simulink model "M4B11_modified_AGC_PI_constant_power"  (R2024b)
settings: Solver=VariableStepAuto  StartTime=0.0  StopTime=100  RelTol=1e-3
InitFcn:
  | clear;
  | load('parameterinit.mat');
  | set_param('M4B11_modified_AGC_PI_constant_power/Python2Sim2','value','[0 0]');
  | acom=100;
  | bcom=50;
  | lam=100;
values from neighbouring files (symbols this model uses):
  ACgirdinit =     [datainit.mat]    (also in parameterinit.mat)
  AVm0 = [11.3576294988 11.3576294988]    [datainit.mat]    (also in parameterinit.mat)
  commun = [1 1 1 0]    [datainit.mat]    (also in initAll.m = [1,1,1,0]; parameterinit.mat)
  DataDelay = [0  0; 0  0; 0  0; 0  0]    [datainit.mat]    (also in initAll.m = 0.0*DataDelay; parameterinit.mat)
  ESinit =     [datainit.mat]    (also in parameterinit.mat)
  fB = 50    [datainit.mat]    (also in initAll.m; parameterinit.mat)
  Geninit =     [datainit.mat]    (also in initAll.m = Generator_init(opdata,SynMach_in_gidx); parameterinit.mat)
  SgridB = 100    [datainit.mat]    (also in initAll.m = resultsac.baseMVA; parameterinit.mat)
  wB = 314.159265359    [datainit.mat]    (also in initAll.m; parameterinit.mat)
  Windinit =     [datainit.mat]    (also in parameterinit.mat)
undefined symbols (not defined in the file or in its folder): c1, c2, c3, c4, c5, c6, cp_nom, lambda_nom, Loadinit, P_wind_base, Pelec_base, Pnom
libraries: spsBistableLib x9, slpidlib x2, simulink_extras x2
(part 3 of 5)

== system M4B11_modified_AGC_PI_constant_power/ES1/ control1 ==
  usdq : Inport
  isdq : Inport  Port=2
  delta : Inport  Port=3
  Enable : EnablePort
  Add : Sum  Inputs=|-+
  Add2 : Sum  Inputs=|-+
  Add3 : Sum
  Add4 : Sum  Inputs=-+
  Add6 : Sum  Inputs=|++
  Add7 : Sum  Inputs=+-
  Complex to Magnitude-Angle : ComplexToMagnitudeAngle
  Complex to Real-Imag1 : ComplexToRealImag
  Constant : Constant
  Constant1 : Constant  Value=usd0
  Constant2 : Constant  Value=0
  Constant3 : Constant  Value=Q0
  Constant4 : Constant
  Demux : Demux  Outputs=2
  Demux1 : Demux  Outputs=2
  Gain : Gain  Gain=0.01
  Gain1 : Gain  Gain=-1
  K5 : Gain  Gain=Lpr  SaturateOnIntegerOverflow=on  OutDataTypeStr=Inherit: Same as input  ParamDataTypeStr=Inherit: Same as input
  K6 : Gain  Gain=Lpr  SaturateOnIntegerOverflow=on  OutDataTypeStr=Inherit: Same as input  ParamDataTypeStr=Inherit: Same as input
  Magnitude-Angle to Complex : MagnitudeAngleToComplex
  Product{1,4..6} (4 alike) : Product  RndMeth=Zero
  Real-Imag to Complex : RealImagToComplex
  Scope : Scope
  Scope1 : Scope
  Scope2 : Scope  NumInputPorts=2
  Scope3 : Scope  NumInputPorts=2
  Scope7 : Scope  NumInputPorts=2
  Sum : Sum  Inputs=|+-
  Sum2 : Sum  Inputs=|+-  SaturateOnIntegerOverflow=on
  Sum23 : Sum  Inputs=|+-  SaturateOnIntegerOverflow=on
  Sum9 : Sum  Inputs=|+-  SaturateOnIntegerOverflow=on
  control_AC_voltage : Subsystem  VariantControl=VSC1q_Variant2
  control_AC_voltage1 : Subsystem  VariantControl=VSC1q_Variant2
  in_D_PI : Subsystem  mask{KP_=KpId_VSC_A, KI_=KiId_VSC_A, Upper_limit=inf, Lower_limit=-inf, Upper_saturation_limit=inf, Lower_saturation_limit=-inf, integrator_init=Md_A_0}
      mask prompts: KP_ "比例系数P"; KI_ "积分系数I"; Upper_limit "限幅上限"; Lower_limit "限幅下限"; Upper_saturation_limit "积分饱和上限"; Lower_saturation_limit "积分饱和下限"; integrator_init "积分初始值"
      mask DialogControl Container4 Prompt: 控制参数
      mask DialogControl Container5 Prompt: 初始值
      mask Display: disp('PI')
  in_Q_PI : Subsystem  mask{KP_=KpIq_VSC_A, KI_=KiIq_VSC_A, Upper_limit=inf, Lower_limit=-inf, Upper_saturation_limit=inf, Lower_saturation_limit=-inf, integrator_init=Mq_A_0}
      mask prompts: KP_ "比例系数P"; KI_ "积分系数I"; Upper_limit "限幅上限"; Lower_limit "限幅下限"; Upper_saturation_limit "积分饱和上限"; Lower_saturation_limit "积分饱和下限"; integrator_init "积分初始值"
      mask DialogControl Container4 Prompt: 控制参数
      mask DialogControl Container5 Prompt: 初始值
      mask Display: disp('PI')
  ucx : Outport
  ucy : Outport  Port=2
  wires:
  Magnitude-Angle to Complex/1 -> Complex to Real-Imag1/1
  Add/1 -> Real-Imag to Complex/2
  Add2/1 -> Real-Imag to Complex/1
  delta/1 -> Add6/2
  Add6/1 -> Magnitude-Angle to Complex/2
  Complex to Magnitude-Angle/2 -> Add6/1
  Sum9/1 -> in_D_PI/1(In1)
  K5/1 -> Add3/1
  [usd] -> Add3/2
  Add3/1 -> Add2/2
  in_D_PI/1(Out1) -> Add2/1
  Constant/1 -> Product4/2
  [isq] -> Product4/1
  [isd] -> Scope7/2, Sum9/2
  Product4/1 -> K5/1
  Demux1/1 -> [isd]
  Demux/1 -> [usd]
  Demux1/2 -> [isq]
  Demux/2 -> [usq]
  isdq/1 -> Demux1/1
  usdq/1 -> Demux/1
  [usq] -> Add4/2
  K6/1 -> Add4/1
  in_Q_PI/1(Out1) -> Add/1
  Sum23/1 -> in_Q_PI/1(In1)
  [isd] -> Product1/1
  [isq] -> Sum23/2, Scope3/2
  Product1/1 -> K6/1
  Constant4/1 -> Product1/2
  Add4/1 -> Add/2
  Real-Imag to Complex/1 -> Complex to Magnitude-Angle/1
  Complex to Magnitude-Angle/1 -> Magnitude-Angle to Complex/1
  Complex to Real-Imag1/1 -> ucx/1
  Complex to Real-Imag1/2 -> ucy/1
  [usd] -> Scope1/1, control_AC_voltage/1(usd)
  control_AC_voltage/1(isdref) -> Scope7/1, Sum9/1
  [isq] -> Product5/2
  Product5/1 -> Add7/2
  [usd] -> Product5/1
  [isd] -> Product6/2
  Product6/1 -> Add7/1
  [usq] -> Product6/1
  Gain/1 -> Sum/2
  control_AC_voltage1/1(isqref) -> Scope3/1, Sum23/1
  [usq] -> Scope2/1, control_AC_voltage1/1(usq)
  Constant2/1 -> Scope2/2, control_AC_voltage1/2(usqref)
  Add7/1 -> Scope/1, Gain1/1
  Sum2/1 -> Gain/1
  Constant3/1 -> Sum2/2
  Gain1/1 -> Sum2/1
  Sum/1 -> control_AC_voltage/2(usdref)
  Constant1/1 -> Sum/1

== system M4B11_modified_AGC_PI_constant_power/ES1/in_D_PI ==
  In1 : Inport
  Ki : Gain  Gain=KI_  SaturateOnIntegerOverflow=on  OutDataTypeStr=Inherit: Same as input  ParamDataTypeStr=Inherit: Same as input
  Kp : Gain  Gain=KP_  SaturateOnIntegerOverflow=on  OutDataTypeStr=Inherit: Same as input  ParamDataTypeStr=Inherit: Same as input
  Saturation2 : Saturate  UpperLimit=Upper_limit  LowerLimit=Lower_limit
  Sum12 : Sum  SaturateOnIntegerOverflow=on
  integrator : Integrator  InitialCondition=integrator_init  LimitOutput=on  UpperSaturationLimit=Upper_saturation_limit  LowerSaturationLimit=Lower_saturation_limit
  Out1 : Outport
  wires:
  In1/1 -> Ki/1, Kp/1
  Kp/1 -> Sum12/2
  Ki/1 -> integrator/1
  integrator/1 -> Sum12/1
  Saturation2/1 -> Out1/1
  Sum12/1 -> Saturation2/1

== system M4B11_modified_AGC_PI_constant_power/ES1/output ==
  is_xy : Inport
  Pe : Inport  Port=2
  Brecx : Constant  Value=0
  Brecy : Constant  Value=0
  Bus Creator : BusCreator  Inputs=4
  Constant : Constant
  Gain : Gain  Gain=SvscB./SgridB
  Gain1 : Gain  Gain=-1
  Gain2 : Gain  Gain=-1
  Gain6 : Gain
  Grecx : Constant  Value=0
  Grecy : Constant  Value=0
  Mux3 : Mux
  Sum : Sum  Inputs=|++
  m : Outport
  isxy : Outport  Port=2
  GBxy : Outport  Port=3
  wires:
  Bus Creator/1 -> m/1
  Gain6/1 -> GBxy/1, Bus Creator/4  "GBxy"
  Mux3/1 -> Gain6/1
  Grecx/1 -> Mux3/1
  Brecx/1 -> Mux3/3
  Grecy/1 -> Mux3/2
  Brecy/1 -> Mux3/4
  Gain1/1 -> isxy/1, Bus Creator/1  "is_xy"
  Gain2/1 -> Bus Creator/2  "Pe"
  Gain/1 -> Gain1/1  "is_xy"
  Pe/1 -> Gain2/1  "Pe"
  [WreES1] -> Sum/1  "Pe"
  Constant/1 -> Sum/2
  Sum/1 -> Bus Creator/3  "w"
  is_xy/1 -> Gain/1

== system M4B11_modified_AGC_PI_constant_power/ES1/xy->dq ==
  Ixy : Inport
  Theta : Inport  Port=2
  Complex to Magnitude-Angle : ComplexToMagnitudeAngle
  Complex to Real-Imag : ComplexToRealImag
  Demux1 : Demux  Outputs=2
      settings: DisplayOption=none
  Magnitude-Angle to Complex : MagnitudeAngleToComplex
  Mux : Mux  Inputs=2
  Real-Imag to Complex : RealImagToComplex
  Scope : Scope
  Scope1 : Scope
  Sum1 : Sum  Inputs=|+-  SaturateOnIntegerOverflow=on
  Idq : Outport
  wires:
  Complex to Magnitude-Angle/1 -> Magnitude-Angle to Complex/1
  Theta/1 -> Sum1/2
  Complex to Magnitude-Angle/2 -> Sum1/1, Scope1/1
  Demux1/1 -> Real-Imag to Complex/1
  Complex to Real-Imag/2 -> Mux/2  "Iq"
  Mux/1 -> Idq/1
  Complex to Real-Imag/1 -> Mux/1  "Id"
  Magnitude-Angle to Complex/1 -> Complex to Real-Imag/1
  Sum1/1 -> Magnitude-Angle to Complex/2, Scope/1
  Demux1/2 -> Real-Imag to Complex/2
  Real-Imag to Complex/1 -> Complex to Magnitude-Angle/1
  Ixy/1 -> Demux1/1

== system M4B11_modified_AGC_PI_constant_power/ES2/ control1 ==
  usdq : Inport
  isdq : Inport  Port=2
  delta : Inport  Port=3
  Enable : EnablePort
  Add : Sum  Inputs=|-+
  Add2 : Sum  Inputs=|-+
  Add3 : Sum
  Add4 : Sum  Inputs=-+
  Add6 : Sum  Inputs=|++
  Add7 : Sum  Inputs=+-
  Complex to Magnitude-Angle : ComplexToMagnitudeAngle
  Complex to Real-Imag1 : ComplexToRealImag
  Constant : Constant
  Constant1 : Constant  Value=usd0
  Constant2 : Constant  Value=0
  Constant3 : Constant  Value=Q0
  Constant4 : Constant
  Demux : Demux  Outputs=2
  Demux1 : Demux  Outputs=2
  Gain : Gain  Gain=0.01
  Gain1 : Gain  Gain=-1
  K5 : Gain  Gain=Lpr  SaturateOnIntegerOverflow=on  OutDataTypeStr=Inherit: Same as input  ParamDataTypeStr=Inherit: Same as input
  K6 : Gain  Gain=Lpr  SaturateOnIntegerOverflow=on  OutDataTypeStr=Inherit: Same as input  ParamDataTypeStr=Inherit: Same as input
  Magnitude-Angle to Complex : MagnitudeAngleToComplex
  Product{1,4..6} (4 alike) : Product  RndMeth=Zero
  Real-Imag to Complex : RealImagToComplex
  Scope{,1..2,7} (4 alike) : Scope
  Sum : Sum  Inputs=|+-
  Sum2 : Sum  Inputs=|+-  SaturateOnIntegerOverflow=on
  Sum23 : Sum  Inputs=|+-  SaturateOnIntegerOverflow=on
  Sum9 : Sum  Inputs=|+-  SaturateOnIntegerOverflow=on
  control_AC_voltage : Subsystem  VariantControl=VSC1q_Variant2
  control_AC_voltage1 : Subsystem  VariantControl=VSC1q_Variant2
  in_D_PI : Subsystem  mask{KP_=KpId_VSC_A, KI_=KiId_VSC_A, Upper_limit=inf, Lower_limit=-inf, Upper_saturation_limit=inf, Lower_saturation_limit=-inf, integrator_init=Md_A_0}
      mask prompts: KP_ "比例系数P"; KI_ "积分系数I"; Upper_limit "限幅上限"; Lower_limit "限幅下限"; Upper_saturation_limit "积分饱和上限"; Lower_saturation_limit "积分饱和下限"; integrator_init "积分初始值"
      mask DialogControl Container4 Prompt: 控制参数
      mask DialogControl Container5 Prompt: 初始值
      mask Display: disp('PI')
  in_Q_PI : Subsystem  mask{KP_=KpIq_VSC_A, KI_=KiIq_VSC_A, Upper_limit=inf, Lower_limit=-inf, Upper_saturation_limit=inf, Lower_saturation_limit=-inf, integrator_init=Mq_A_0}
      mask prompts: KP_ "比例系数P"; KI_ "积分系数I"; Upper_limit "限幅上限"; Lower_limit "限幅下限"; Upper_saturation_limit "积分饱和上限"; Lower_saturation_limit "积分饱和下限"; integrator_init "积分初始值"
      mask DialogControl Container4 Prompt: 控制参数
      mask DialogControl Container5 Prompt: 初始值
      mask Display: disp('PI')
  ucx : Outport
  ucy : Outport  Port=2
  wires:
  Magnitude-Angle to Complex/1 -> Complex to Real-Imag1/1
  Add/1 -> Real-Imag to Complex/2
  Add2/1 -> Real-Imag to Complex/1
  delta/1 -> Add6/2
  Add6/1 -> Magnitude-Angle to Complex/2
  Complex to Magnitude-Angle/2 -> Add6/1
  Sum9/1 -> in_D_PI/1(In1)
  K5/1 -> Add3/1
  [usd] -> Add3/2
  Add3/1 -> Add2/2
  in_D_PI/1(Out1) -> Add2/1
  Constant/1 -> Product4/2
  [isq] -> Product4/1
  [isd] -> Sum9/2
  Product4/1 -> K5/1
  Demux1/1 -> [isd]
  Demux/1 -> [usd]
  Demux1/2 -> [isq]
  Demux/2 -> [usq]
  isdq/1 -> Demux1/1
  usdq/1 -> Demux/1
  [usq] -> Add4/2
  K6/1 -> Add4/1
  in_Q_PI/1(Out1) -> Add/1
  Sum23/1 -> in_Q_PI/1(In1)
  [isd] -> Product1/1
  [isq] -> Sum23/2
  Product1/1 -> K6/1
  Constant4/1 -> Product1/2
  Add4/1 -> Add/2
  Real-Imag to Complex/1 -> Complex to Magnitude-Angle/1
  Complex to Magnitude-Angle/1 -> Magnitude-Angle to Complex/1
  Complex to Real-Imag1/1 -> ucx/1
  Complex to Real-Imag1/2 -> ucy/1
  [usd] -> Scope1/1, control_AC_voltage/1(usd)
  control_AC_voltage/1(isdref) -> Scope7/1, Sum9/1
  [isq] -> Product5/2
  Product5/1 -> Add7/2
  [usd] -> Product5/1
  [isd] -> Product6/2
  Product6/1 -> Add7/1
  [usq] -> Product6/1
  Gain/1 -> Sum/2
  control_AC_voltage1/1(isqref) -> Sum23/1
  [usq] -> Scope2/1, control_AC_voltage1/1(usq)
  Constant2/1 -> control_AC_voltage1/2(usqref)
  Add7/1 -> Scope/1, Gain1/1
  Sum2/1 -> Gain/1
  Constant3/1 -> Sum2/2
  Gain1/1 -> Sum2/1
  Sum/1 -> control_AC_voltage/2(usdref)
  Constant1/1 -> Sum/1

== system M4B11_modified_AGC_PI_constant_power/ES2/output ==
  is_xy : Inport
  Pe : Inport  Port=2
  Brecx : Constant  Value=0
  Brecy : Constant  Value=0
  Bus Creator : BusCreator  Inputs=4
  Constant : Constant
  Gain : Gain  Gain=SvscB./SgridB
  Gain1 : Gain  Gain=-1
  Gain2 : Gain  Gain=-1
  Gain6 : Gain
  Grecx : Constant  Value=0
  Grecy : Constant  Value=0
  Mux3 : Mux
  Sum : Sum  Inputs=|++
  m : Outport
  isxy : Outport  Port=2
  GBxy : Outport  Port=3
  wires:
  Bus Creator/1 -> m/1
  Gain6/1 -> GBxy/1, Bus Creator/4  "GBxy"
  Mux3/1 -> Gain6/1
  Grecx/1 -> Mux3/1
  Brecx/1 -> Mux3/3
  Grecy/1 -> Mux3/2
  Brecy/1 -> Mux3/4
  Gain1/1 -> isxy/1, Bus Creator/1  "is_xy"
  Gain2/1 -> Bus Creator/2  "Pe"
  Gain/1 -> Gain1/1  "is_xy"
  Pe/1 -> Gain2/1  "Pe"
  Constant/1 -> Sum/2
  [WreES2] -> Sum/1  "Pe"
  Sum/1 -> Bus Creator/3  "w"
  is_xy/1 -> Gain/1

== system M4B11_modified_AGC_PI_constant_power/ES2/xy->dq ==
  Ixy : Inport
  Theta : Inport  Port=2
  Complex to Magnitude-Angle : ComplexToMagnitudeAngle
  Complex to Real-Imag : ComplexToRealImag
  Demux1 : Demux  Outputs=2
      settings: DisplayOption=none
  Magnitude-Angle to Complex : MagnitudeAngleToComplex
  Mux : Mux  Inputs=2
  Real-Imag to Complex : RealImagToComplex
  Scope : Scope
  Scope1 : Scope
  Sum1 : Sum  Inputs=|+-  SaturateOnIntegerOverflow=on
  Idq : Outport
  wires:
  Complex to Magnitude-Angle/1 -> Magnitude-Angle to Complex/1
  Theta/1 -> Sum1/2
  Complex to Magnitude-Angle/2 -> Sum1/1, Scope1/1
  Demux1/1 -> Real-Imag to Complex/1
  Complex to Real-Imag/2 -> Mux/2  "Iq"
  Mux/1 -> Idq/1
  Complex to Real-Imag/1 -> Mux/1  "Id"
  Magnitude-Angle to Complex/1 -> Complex to Real-Imag/1
  Sum1/1 -> Magnitude-Angle to Complex/2, Scope/1
  Demux1/2 -> Real-Imag to Complex/2
  Real-Imag to Complex/1 -> Complex to Magnitude-Angle/1
  Ixy/1 -> Demux1/1

== system M4B11_modified_AGC_PI_constant_power/ES3/ control1 ==
  usdq : Inport
  isdq : Inport  Port=2
  delta : Inport  Port=3
  Enable : EnablePort
  Add : Sum  Inputs=|-+
  Add2 : Sum  Inputs=|-+
  Add3 : Sum
  Add4 : Sum  Inputs=-+
  Add6 : Sum  Inputs=|++
  Add7 : Sum  Inputs=+-
  Complex to Magnitude-Angle : ComplexToMagnitudeAngle
  Complex to Real-Imag1 : ComplexToRealImag
  Constant : Constant
  Constant1 : Constant  Value=usd0
  Constant2 : Constant  Value=0
  Constant3 : Constant  Value=Q0
  Constant4 : Constant
  Demux : Demux  Outputs=2
  Demux1 : Demux  Outputs=2
  Gain : Gain  Gain=0.01
  Gain1 : Gain  Gain=-1
  K5 : Gain  Gain=Lpr  SaturateOnIntegerOverflow=on  OutDataTypeStr=Inherit: Same as input  ParamDataTypeStr=Inherit: Same as input
  K6 : Gain  Gain=Lpr  SaturateOnIntegerOverflow=on  OutDataTypeStr=Inherit: Same as input  ParamDataTypeStr=Inherit: Same as input
  Magnitude-Angle to Complex : MagnitudeAngleToComplex
  Product{1,4..6} (4 alike) : Product  RndMeth=Zero
  Real-Imag to Complex : RealImagToComplex
  Scope{,1..2,7} (4 alike) : Scope
  Sum : Sum  Inputs=|+-
  Sum2 : Sum  Inputs=|+-  SaturateOnIntegerOverflow=on
  Sum23 : Sum  Inputs=|+-  SaturateOnIntegerOverflow=on
  Sum9 : Sum  Inputs=|+-  SaturateOnIntegerOverflow=on
  control_AC_voltage : Subsystem  VariantControl=VSC1q_Variant2
  control_AC_voltage1 : Subsystem  VariantControl=VSC1q_Variant2
  in_D_PI : Subsystem  mask{KP_=KpId_VSC_A, KI_=KiId_VSC_A, Upper_limit=inf, Lower_limit=-inf, Upper_saturation_limit=inf, Lower_saturation_limit=-inf, integrator_init=Md_A_0}
      mask prompts: KP_ "比例系数P"; KI_ "积分系数I"; Upper_limit "限幅上限"; Lower_limit "限幅下限"; Upper_saturation_limit "积分饱和上限"; Lower_saturation_limit "积分饱和下限"; integrator_init "积分初始值"
      mask DialogControl Container4 Prompt: 控制参数
      mask DialogControl Container5 Prompt: 初始值
      mask Display: disp('PI')
  in_Q_PI : Subsystem  mask{KP_=KpIq_VSC_A, KI_=KiIq_VSC_A, Upper_limit=inf, Lower_limit=-inf, Upper_saturation_limit=inf, Lower_saturation_limit=-inf, integrator_init=Mq_A_0}
      mask prompts: KP_ "比例系数P"; KI_ "积分系数I"; Upper_limit "限幅上限"; Lower_limit "限幅下限"; Upper_saturation_limit "积分饱和上限"; Lower_saturation_limit "积分饱和下限"; integrator_init "积分初始值"
      mask DialogControl Container4 Prompt: 控制参数
      mask DialogControl Container5 Prompt: 初始值
      mask Display: disp('PI')
  ucx : Outport
  ucy : Outport  Port=2
  wires:
  Magnitude-Angle to Complex/1 -> Complex to Real-Imag1/1
  Add/1 -> Real-Imag to Complex/2
  Add2/1 -> Real-Imag to Complex/1
  delta/1 -> Add6/2
  Add6/1 -> Magnitude-Angle to Complex/2
  Complex to Magnitude-Angle/2 -> Add6/1
  Sum9/1 -> in_D_PI/1(In1)
  K5/1 -> Add3/1
  [usd] -> Add3/2
  Add3/1 -> Add2/2
  in_D_PI/1(Out1) -> Add2/1
  Constant/1 -> Product4/2
  [isq] -> Product4/1
  [isd] -> Sum9/2
  Product4/1 -> K5/1
  Demux1/1 -> [isd]
  Demux/1 -> [usd]
  Demux1/2 -> [isq]
  Demux/2 -> [usq]
  isdq/1 -> Demux1/1
  usdq/1 -> Demux/1
  [usq] -> Add4/2
  K6/1 -> Add4/1
  in_Q_PI/1(Out1) -> Add/1
  Sum23/1 -> in_Q_PI/1(In1)
  [isd] -> Product1/1
  [isq] -> Sum23/2
  Product1/1 -> K6/1
  Constant4/1 -> Product1/2
  Add4/1 -> Add/2
  Real-Imag to Complex/1 -> Complex to Magnitude-Angle/1
  Complex to Magnitude-Angle/1 -> Magnitude-Angle to Complex/1
  Complex to Real-Imag1/1 -> ucx/1
  Complex to Real-Imag1/2 -> ucy/1
  [usd] -> Scope1/1, control_AC_voltage/1(usd)
  control_AC_voltage/1(isdref) -> Scope7/1, Sum9/1
  [isq] -> Product5/2
  Product5/1 -> Add7/2
  [usd] -> Product5/1
  [isd] -> Product6/2
  Product6/1 -> Add7/1
  [usq] -> Product6/1
  Gain/1 -> Sum/2
  control_AC_voltage1/1(isqref) -> Sum23/1
  [usq] -> Scope2/1, control_AC_voltage1/1(usq)
  Constant2/1 -> control_AC_voltage1/2(usqref)
  Add7/1 -> Scope/1, Gain1/1
  Sum2/1 -> Gain/1
  Constant3/1 -> Sum2/2
  Gain1/1 -> Sum2/1
  Sum/1 -> control_AC_voltage/2(usdref)
  Constant1/1 -> Sum/1

== system M4B11_modified_AGC_PI_constant_power/ES3/in_D_PI ==
  In1 : Inport
  Ki : Gain  Gain=KI_  SaturateOnIntegerOverflow=on  OutDataTypeStr=Inherit: Same as input  ParamDataTypeStr=Inherit: Same as input
  Kp : Gain  Gain=KP_  SaturateOnIntegerOverflow=on  OutDataTypeStr=Inherit: Same as input  ParamDataTypeStr=Inherit: Same as input
  Saturation2 : Saturate  UpperLimit=Upper_limit  LowerLimit=Lower_limit
  Sum12 : Sum  SaturateOnIntegerOverflow=on
  integrator : Integrator  InitialCondition=integrator_init  LimitOutput=on  UpperSaturationLimit=Upper_saturation_limit  LowerSaturationLimit=Lower_saturation_limit
  Out1 : Outport
  wires:
  In1/1 -> Ki/1, Kp/1
  Kp/1 -> Sum12/2
  Ki/1 -> integrator/1
  integrator/1 -> Sum12/1
  Saturation2/1 -> Out1/1
  Sum12/1 -> Saturation2/1

== system M4B11_modified_AGC_PI_constant_power/ES3/output ==
  is_xy : Inport
  Pe : Inport  Port=2
  Brecx : Constant  Value=0
  Brecy : Constant  Value=0
  Bus Creator : BusCreator  Inputs=4
  Constant : Constant
  Gain : Gain  Gain=SvscB./SgridB
  Gain1 : Gain  Gain=-1
  Gain2 : Gain  Gain=-1
  Gain6 : Gain
  Grecx : Constant  Value=0
  Grecy : Constant  Value=0
  Mux3 : Mux
  Sum : Sum  Inputs=|++
  m : Outport
  isxy : Outport  Port=2
  GBxy : Outport  Port=3
  wires:
  Bus Creator/1 -> m/1
  Gain6/1 -> GBxy/1, Bus Creator/4  "GBxy"
  Mux3/1 -> Gain6/1
  Grecx/1 -> Mux3/1
  Brecx/1 -> Mux3/3
  Grecy/1 -> Mux3/2
  Brecy/1 -> Mux3/4
  Gain1/1 -> isxy/1, Bus Creator/1  "is_xy"
  Gain2/1 -> Bus Creator/2  "Pe"
  Gain/1 -> Gain1/1  "is_xy"
  Pe/1 -> Gain2/1  "Pe"
  Constant/1 -> Sum/2
  [WreES3] -> Sum/1  "Pe"
  Sum/1 -> Bus Creator/3  "w"
  is_xy/1 -> Gain/1

== system M4B11_modified_AGC_PI_constant_power/ES3/xy->dq ==
  Ixy : Inport
  Theta : Inport  Port=2
  Complex to Magnitude-Angle : ComplexToMagnitudeAngle
  Complex to Real-Imag : ComplexToRealImag
  Demux1 : Demux  Outputs=2
      settings: DisplayOption=none
  Magnitude-Angle to Complex : MagnitudeAngleToComplex
  Mux : Mux  Inputs=2
  Real-Imag to Complex : RealImagToComplex
  Scope : Scope
  Scope1 : Scope
  Sum1 : Sum  Inputs=|+-  SaturateOnIntegerOverflow=on
  Idq : Outport
  wires:
  Complex to Magnitude-Angle/1 -> Magnitude-Angle to Complex/1
  Theta/1 -> Sum1/2
  Complex to Magnitude-Angle/2 -> Sum1/1, Scope1/1
  Demux1/1 -> Real-Imag to Complex/1
  Complex to Real-Imag/2 -> Mux/2  "Iq"
  Mux/1 -> Idq/1
  Complex to Real-Imag/1 -> Mux/1  "Id"
  Magnitude-Angle to Complex/1 -> Complex to Real-Imag/1
  Sum1/1 -> Magnitude-Angle to Complex/2, Scope/1
  Demux1/2 -> Real-Imag to Complex/2
  Real-Imag to Complex/1 -> Complex to Magnitude-Angle/1
  Ixy/1 -> Demux1/1

== system M4B11_modified_AGC_PI_constant_power/ES4/ control1 ==
  usdq : Inport
  isdq : Inport  Port=2
  delta : Inport  Port=3
  Enable : EnablePort
  Add : Sum  Inputs=|-+
  Add2 : Sum  Inputs=|-+
  Add3 : Sum
  Add4 : Sum  Inputs=-+
  Add6 : Sum  Inputs=|++
  Add7 : Sum  Inputs=+-
  Complex to Magnitude-Angle : ComplexToMagnitudeAngle
  Complex to Real-Imag1 : ComplexToRealImag
  Constant : Constant
  Constant1 : Constant  Value=usd0
  Constant2 : Constant  Value=0
  Constant3 : Constant  Value=Q0
  Constant4 : Constant
  Demux : Demux  Outputs=2
  Demux1 : Demux  Outputs=2
  Gain1 : Gain  Gain=-1
  Gain2 : Gain  Gain=0.01
  K5 : Gain  Gain=Lpr  SaturateOnIntegerOverflow=on  OutDataTypeStr=Inherit: Same as input  ParamDataTypeStr=Inherit: Same as input
  K6 : Gain  Gain=Lpr  SaturateOnIntegerOverflow=on  OutDataTypeStr=Inherit: Same as input  ParamDataTypeStr=Inherit: Same as input
  Magnitude-Angle to Complex : MagnitudeAngleToComplex
  Product{1,4..6} (4 alike) : Product  RndMeth=Zero
  Real-Imag to Complex : RealImagToComplex
  Scope{,1..2,7} (4 alike) : Scope
  Sum : Sum  Inputs=|+-
  Sum2 : Sum  Inputs=|+-  SaturateOnIntegerOverflow=on
  Sum23 : Sum  Inputs=|+-  SaturateOnIntegerOverflow=on
  Sum9 : Sum  Inputs=|+-  SaturateOnIntegerOverflow=on
  control_AC_voltage : Subsystem  VariantControl=VSC1q_Variant2
  control_AC_voltage1 : Subsystem  VariantControl=VSC1q_Variant2
  in_D_PI : Subsystem  mask{KP_=KpId_VSC_A, KI_=KiId_VSC_A, Upper_limit=inf, Lower_limit=-inf, Upper_saturation_limit=inf, Lower_saturation_limit=-inf, integrator_init=Md_A_0}
      mask prompts: KP_ "比例系数P"; KI_ "积分系数I"; Upper_limit "限幅上限"; Lower_limit "限幅下限"; Upper_saturation_limit "积分饱和上限"; Lower_saturation_limit "积分饱和下限"; integrator_init "积分初始值"
      mask DialogControl Container4 Prompt: 控制参数
      mask DialogControl Container5 Prompt: 初始值
      mask Display: disp('PI')
  in_Q_PI : Subsystem  mask{KP_=KpIq_VSC_A, KI_=KiIq_VSC_A, Upper_limit=inf, Lower_limit=-inf, Upper_saturation_limit=inf, Lower_saturation_limit=-inf, integrator_init=Mq_A_0}
      mask prompts: KP_ "比例系数P"; KI_ "积分系数I"; Upper_limit "限幅上限"; Lower_limit "限幅下限"; Upper_saturation_limit "积分饱和上限"; Lower_saturation_limit "积分饱和下限"; integrator_init "积分初始值"
      mask DialogControl Container4 Prompt: 控制参数
      mask DialogControl Container5 Prompt: 初始值
      mask Display: disp('PI')
  ucx : Outport
  ucy : Outport  Port=2
  wires:
  Magnitude-Angle to Complex/1 -> Complex to Real-Imag1/1
  Add/1 -> Real-Imag to Complex/2
  Add2/1 -> Real-Imag to Complex/1
  delta/1 -> Add6/2
  Add6/1 -> Magnitude-Angle to Complex/2
  Complex to Magnitude-Angle/2 -> Add6/1
  Sum9/1 -> in_D_PI/1(In1)
  K5/1 -> Add3/1
  [usd] -> Add3/2
  Add3/1 -> Add2/2
  in_D_PI/1(Out1) -> Add2/1
  Constant/1 -> Product4/2
  [isq] -> Product4/1
  [isd] -> Sum9/2
  Product4/1 -> K5/1
  Demux1/1 -> [isd]
  Demux/1 -> [usd]
  Demux1/2 -> [isq]
  Demux/2 -> [usq]
  isdq/1 -> Demux1/1
  usdq/1 -> Demux/1
  [usq] -> Add4/2
  K6/1 -> Add4/1
  in_Q_PI/1(Out1) -> Add/1
  Sum23/1 -> in_Q_PI/1(In1)
  [isd] -> Product1/1
  [isq] -> Sum23/2
  Product1/1 -> K6/1
  Constant4/1 -> Product1/2
  Add4/1 -> Add/2
  Real-Imag to Complex/1 -> Complex to Magnitude-Angle/1
  Complex to Magnitude-Angle/1 -> Magnitude-Angle to Complex/1
  Complex to Real-Imag1/1 -> ucx/1
  Complex to Real-Imag1/2 -> ucy/1
  [usd] -> Scope1/1, control_AC_voltage/1(usd)
  control_AC_voltage/1(isdref) -> Scope7/1, Sum9/1
  [isq] -> Product5/2
  Product5/1 -> Add7/2
  [usd] -> Product5/1
  [isd] -> Product6/2
  Product6/1 -> Add7/1
  [usq] -> Product6/1
  Gain2/1 -> Sum/2
  control_AC_voltage1/1(isqref) -> Sum23/1
  [usq] -> Scope2/1, control_AC_voltage1/1(usq)
  Constant2/1 -> control_AC_voltage1/2(usqref)
  Add7/1 -> Scope/1, Gain1/1
  Sum2/1 -> Gain2/1
  Constant3/1 -> Sum2/2
  Gain1/1 -> Sum2/1
  Sum/1 -> control_AC_voltage/2(usdref)
  Constant1/1 -> Sum/1

== system M4B11_modified_AGC_PI_constant_power/ES4/output ==
  is_xy : Inport
  Pe : Inport  Port=2
  Brecx : Constant  Value=0
  Brecy : Constant  Value=0
  Bus Creator : BusCreator  Inputs=4
  Constant : Constant
  Gain : Gain  Gain=SvscB./SgridB
  Gain1 : Gain  Gain=-1
  Gain2 : Gain  Gain=-1
  Gain6 : Gain
  Grecx : Constant  Value=0
  Grecy : Constant  Value=0
  Mux3 : Mux
  Sum : Sum  Inputs=|++
  m : Outport
  isxy : Outport  Port=2
  GBxy : Outport  Port=3
  wires:
  Bus Creator/1 -> m/1
  Gain6/1 -> GBxy/1, Bus Creator/4  "GBxy"
  Mux3/1 -> Gain6/1
  Grecx/1 -> Mux3/1
  Brecx/1 -> Mux3/3
  Grecy/1 -> Mux3/2
  Brecy/1 -> Mux3/4
  Gain1/1 -> isxy/1, Bus Creator/1  "is_xy"
  Gain2/1 -> Bus Creator/2  "Pe"
  Gain/1 -> Gain1/1  "is_xy"
  Pe/1 -> Gain2/1  "Pe"
  Constant/1 -> Sum/2
  [WreES4] -> Sum/1  "Pe"
  Sum/1 -> Bus Creator/3  "w"
  is_xy/1 -> Gain/1

== system M4B11_modified_AGC_PI_constant_power/ES4/xy->dq ==
  Ixy : Inport
  Theta : Inport  Port=2
  Complex to Magnitude-Angle : ComplexToMagnitudeAngle
  Complex to Real-Imag : ComplexToRealImag
  Demux1 : Demux  Outputs=2
      settings: DisplayOption=none
  Magnitude-Angle to Complex : MagnitudeAngleToComplex
  Mux : Mux  Inputs=2
  Real-Imag to Complex : RealImagToComplex
  Scope : Scope
  Scope1 : Scope
  Sum1 : Sum  Inputs=|+-  SaturateOnIntegerOverflow=on
  Idq : Outport
  wires:
  Complex to Magnitude-Angle/1 -> Magnitude-Angle to Complex/1
  Theta/1 -> Sum1/2
  Complex to Magnitude-Angle/2 -> Sum1/1, Scope1/1
  Demux1/1 -> Real-Imag to Complex/1
  Complex to Real-Imag/2 -> Mux/2  "Iq"
  Mux/1 -> Idq/1
  Complex to Real-Imag/1 -> Mux/1  "Id"
  Magnitude-Angle to Complex/1 -> Complex to Real-Imag/1
  Sum1/1 -> Magnitude-Angle to Complex/2, Scope/1
  Demux1/2 -> Real-Imag to Complex/2
  Real-Imag to Complex/1 -> Complex to Magnitude-Angle/1
  Ixy/1 -> Demux1/1

== system M4B11_modified_AGC_PI_constant_power/Generator1/Excitation System ==
  note: Ef
  Upss : Inport
  Trip : Inport  Port=2
  Vg : Inport  Port=3
  Constant : Constant  Value=0
  KA : Gain  Gain=Ka  SaturateOnIntegerOverflow=on  OutDataTypeStr=Inherit: Same as input  ParamDataTypeStr=Inherit: Same as input
  Saturation : Saturate  UpperLimit=Efmax  LowerLimit=Efmin
  Scope : Scope  NumInputPorts=2
  Sum4 : Sum  Inputs=+-+  SaturateOnIntegerOverflow=on
  Switch : Switch  Criteria=u2 ~= 0  Threshold=0.5  InputSameDT=off
  Vref : Constant  Value=Vref
  Ef : Outport
  wires:
  Trip/1 -> Switch/2
  Constant/1 -> Switch/1
  Switch/1 -> Ef/1
  Saturation/1 -> Switch/3
  Sum4/1 -> KA/1
  KA/1 -> Saturation/1
  Vg/1 -> Sum4/2, Scope/2
  Upss/1 -> Sum4/3
  Vref/1 -> Scope/1, Sum4/1

== system M4B11_modified_AGC_PI_constant_power/Generator1/Governor ==
  w : Inport
  Trip : Inport  Port=2
  CT : Constant  Value=0
  Constant : Constant  Value=0
  Gain1 : Gain  Gain=1/R  SaturateOnIntegerOverflow=on  OutDataTypeStr=Inherit: Same as input  ParamDataTypeStr=Inherit: Same as input
  Saturation : Saturate  UpperLimit=dPmax  LowerLimit=dPmin
  Sum3 : Sum  Inputs=|+-  SaturateOnIntegerOverflow=on
  Switch : Switch  Threshold=0.5  InputSameDT=off
  Switch1 : Switch  Criteria=u2 ~= 0  Threshold=0.5  InputSameDT=off
  Transfer Fcn1 : TransferFcn  Denominator=[Ts_G 1]
  Transfer Fcn2 : TransferFcn  Numerator=[T3_G 1]  Denominator=[Tc_G 1]
  Transfer Fcn3 : TransferFcn  Numerator=[T4_G 1]  Denominator=[T5_G 1]
  w1 : Constant  Value=S_Gov
  wref : Constant
  dPm : Outport
  wires:
  Constant/1 -> Switch1/1
  Switch/1 -> Switch1/3
  Trip/1 -> Switch1/2
  Switch1/1 -> dPm/1
  CT/1 -> Switch/3
  w1/1 -> Switch/2
  wref/1 -> Sum3/1
  w/1 -> Sum3/2
  Saturation/1 -> Switch/1
  Sum3/1 -> Gain1/1
  Gain1/1 -> Transfer Fcn1/1
  Transfer Fcn1/1 -> Transfer Fcn2/1
  Transfer Fcn2/1 -> Transfer Fcn3/1
  Transfer Fcn3/1 -> Saturation/1

== system M4B11_modified_AGC_PI_constant_power/Generator1/Machine Equations  ==
  note: Idg
  note: Iqg
  delta : Inport
  Vgxy : Inport  Port=2
  Ef : Inport  Port=3
  Trip : Inport  Port=4
  Demux : Demux  Outputs=2
  Demux1 : Demux  Outputs=2
  Fcn1 : Fcn  Expr=u(1)*u(3)+u(2)*u(4)
  Fcn2 : Fcn  Expr=(u(3)-u(2))/Xd11
  Fcn3 : Fcn  Expr=(u(1)-u(4))/Xq11
  Fcn4 : Fcn  Expr=u(2)*u(3)-u(1)*u(4)
  Fcn6 : Fcn  Expr=sqrt(u(1)^2+u(2)^2)
  Interface : Subsystem
  Mux1 : Mux  Inputs=2
  Mux2 : Mux  Inputs=2
  Mux3 : Mux  Inputs=2
  Qe : Scope
  Scope{,1..3} (4 alike) : Scope
  Transient Equations : Subsystem
  Pe : Outport
  Igxy1 : Outport  Port=2
  GBxy : Outport  Port=3
  Vg : Outport  Port=4
  wires:
  Fcn3/1 -> Mux3/2
  Fcn2/1 -> Mux3/1
  Mux3/1 -> Demux1/1, Mux2/2, Transient Equations/1(Idqg)
  Interface/1(Vdqg) -> Demux/1, Mux2/1, Fcn6/1, Mux1/1
  Mux1/1 -> Fcn2/1, Fcn3/1
  Mux2/1 -> Fcn1/1, Fcn4/1
  Ef/1 -> Transient Equations/2(Ef)
  Fcn1/1 -> Pe/1
  Fcn6/1 -> Vg/1
  Fcn4/1 -> Qe/1
  delta/1 -> Interface/1(delta)
  Vgxy/1 -> Interface/2(Vgxy)
  Interface/2(Igxy1) -> Igxy1/1
  Interface/3(GBxy) -> GBxy/1
  Transient Equations/1(Eqd'') -> Mux1/2, Interface/3(Eqd'')
  Demux/1 -> Scope1/1
  Demux1/1 -> Scope/1
  Demux/2 -> Scope2/1
  Demux1/2 -> Scope3/1
  Trip/1 -> [Trip]
  [Trip] -> Transient Equations/3(Trip)

== system M4B11_modified_AGC_PI_constant_power/Generator1/Mechanical DE ==
  Pe : Inport
  dPm : Inport  Port=2
  Trip : Inport  Port=3
  Constant1 : Constant  Value=0
  Constant2 : Constant  Value=0
  Gain : Gain  Gain=wB  SaturateOnIntegerOverflow=on  OutDataTypeStr=Inherit: Same as input  ParamDataTypeStr=Inherit: Same as input
  Gain1 : Gain  Gain=1/H  SaturateOnIntegerOverflow=on  OutDataTypeStr=Inherit: Same as input  ParamDataTypeStr=Inherit: Same as input
  Gain2 : Gain  Gain=D  SaturateOnIntegerOverflow=on  OutDataTypeStr=Inherit: Same as input  ParamDataTypeStr=Inherit: Same as input
  Gain5 : Gain  Gain=180/pi  SaturateOnIntegerOverflow=on  OutDataTypeStr=Inherit: Same as input  ParamDataTypeStr=Inherit: Same as input
  Int1 : Integrator  InitialCondition=delta0
  Int2 : Integrator  InitialCondition=w0
  Pm : Constant  Value=Pm0
  Scope2 : Scope
  Scope4 : Scope
  Scope8 : Scope
  Sum2 : Sum  Inputs=-+-+  SaturateOnIntegerOverflow=on
  Sum3 : Sum  Inputs=|+-  SaturateOnIntegerOverflow=on
  Switch{1..4} (4 alike) : Switch  Criteria=u2 ~= 0  Threshold=0.5  InputSameDT=off
  w0 : Constant
  delta : Outport
  w : Outport  Port=2
  wires:
  [Trip] -> Switch3/2, Switch2/2
  Constant1/1 -> Switch3/1, Switch2/1
  Switch3/1 -> Scope4/1, Sum3/1, w/1
  Int2/1 -> Switch3/3
  Switch2/1 -> Int2/1
  Gain1/1 -> Switch2/3
  Trip/1 -> [Trip]
  [Trip] -> Switch1/2, Switch4/2
  Constant2/1 -> Switch4/1, Switch1/1
  Switch4/1 -> delta/1, Scope2/1, Gain5/1
  Int1/1 -> Switch4/3
  Switch1/1 -> Int1/1
  Gain/1 -> Switch1/3
  Gain5/1 -> Scope8/1
  w0/1 -> Sum3/2
  Sum3/1 -> Gain2/1, Gain/1
  Pm/1 -> Sum2/2
  Gain2/1 -> Sum2/1
  Sum2/1 -> Gain1/1
  Pe/1 -> Sum2/3
  dPm/1 -> Sum2/4

== system M4B11_modified_AGC_PI_constant_power/Generator1/Output ==
  Igxy1in : Inport
  GBxyin : Inport  Port=2
  deltain : Inport  Port=3
  Pein : Inport  Port=4
  fin : Inport  Port=5
  Vg : Inport  Port=6
  Bus Creator : BusCreator  Inputs=6
  m : Outport
  Igxy1 : Outport  Port=2
  GBxy : Outport  Port=3
  wires:
  Bus Creator/1 -> m/1
  Igxy1in/1 -> Igxy1/1, Bus Creator/1  "Igxy1"
  GBxyin/1 -> GBxy/1, Bus Creator/2  "GBxy"
  deltain/1 -> Bus Creator/3  "delta"
  Pein/1 -> Bus Creator/4  "Pe"
  fin/1 -> Bus Creator/5  "f"
  Vg/1 -> Bus Creator/6  "Vg"

== system M4B11_modified_AGC_PI_constant_power/Generator1/PSS1 ==
  w : Inport
  Trip : Inport  Port=2
  CT : Constant  Value=0
  Constant : Constant  Value=0
  Gain : Gain  Gain=Kpss  SaturateOnIntegerOverflow=on  OutDataTypeStr=Inherit: Same as input  ParamDataTypeStr=Inherit: Same as input
  Saturation : Saturate  UpperLimit=Upmax  LowerLimit=Upmin
  Sum3 : Sum  Inputs=|+-  SaturateOnIntegerOverflow=on
  Switch : Switch  Threshold=0.5  InputSameDT=off
  Switch1 : Switch  Threshold=0.5  InputSameDT=off
  Transfer Fcn : TransferFcn  Numerator=[Tw_P 0]  Denominator=[Tw_P 1]
  Transfer Fcn1 : TransferFcn  Numerator=[T1_P 1]  Denominator=[T2_P 1]
  Transfer Fcn2 : TransferFcn  Numerator=[T3_P 1]  Denominator=[T4_P 1]
  w0 : Constant
  w1 : Constant  Value=S_PSS
  Upss : Outport
  wires:
  Constant/1 -> Switch1/1
  Trip/1 -> Switch1/2
  Switch1/1 -> Upss/1
  Switch/1 -> Switch1/3
  Transfer Fcn/1 -> Transfer Fcn1/1
  Gain/1 -> Transfer Fcn/1
  w1/1 -> Switch/2
  CT/1 -> Switch/3
  Saturation/1 -> Switch/1
  Sum3/1 -> Gain/1
  Transfer Fcn2/1 -> Saturation/1
  Transfer Fcn1/1 -> Transfer Fcn2/1
  w/1 -> Sum3/1
  w0/1 -> Sum3/2

== system M4B11_modified_AGC_PI_constant_power/Generator2/Excitation System ==
  note: Ef
  Upss : Inport
  Trip : Inport  Port=2
  Vg : Inport  Port=3
  Constant : Constant  Value=0
  KA : Gain  Gain=Ka  SaturateOnIntegerOverflow=on  OutDataTypeStr=Inherit: Same as input  ParamDataTypeStr=Inherit: Same as input
  Saturation : Saturate  UpperLimit=Efmax  LowerLimit=Efmin
  Scope : Scope  NumInputPorts=2
  Sum4 : Sum  Inputs=+-+  SaturateOnIntegerOverflow=on
  Switch : Switch  Criteria=u2 ~= 0  Threshold=0.5  InputSameDT=off
  Vref : Constant  Value=Vref
  Ef : Outport
  wires:
  Trip/1 -> Switch/2
  Constant/1 -> Switch/1
  Switch/1 -> Ef/1
  Saturation/1 -> Switch/3
  Sum4/1 -> KA/1
  KA/1 -> Saturation/1
  Vg/1 -> Sum4/2, Scope/2
  Upss/1 -> Sum4/3
  Vref/1 -> Scope/1, Sum4/1

== system M4B11_modified_AGC_PI_constant_power/Generator2/Governor ==
  w : Inport
  Trip : Inport  Port=2
  CT : Constant  Value=0
  Constant : Constant  Value=0
  Gain1 : Gain  Gain=1/R  SaturateOnIntegerOverflow=on  OutDataTypeStr=Inherit: Same as input  ParamDataTypeStr=Inherit: Same as input
  Saturation : Saturate  UpperLimit=dPmax  LowerLimit=dPmin
  Sum3 : Sum  Inputs=|+-  SaturateOnIntegerOverflow=on
  Switch : Switch  Threshold=0.5  InputSameDT=off
  Switch1 : Switch  Criteria=u2 ~= 0  Threshold=0.5  InputSameDT=off
  Transfer Fcn1 : TransferFcn  Denominator=[Ts_G 1]
  Transfer Fcn2 : TransferFcn  Numerator=[T3_G 1]  Denominator=[Tc_G 1]
  Transfer Fcn3 : TransferFcn  Numerator=[T4_G 1]  Denominator=[T5_G 1]
  w1 : Constant  Value=S_Gov
  wref : Constant
  dPm : Outport
  wires:
  Constant/1 -> Switch1/1
  Switch/1 -> Switch1/3
  Trip/1 -> Switch1/2
  Switch1/1 -> dPm/1
  CT/1 -> Switch/3
  w1/1 -> Switch/2
  wref/1 -> Sum3/1
  w/1 -> Sum3/2
  Saturation/1 -> Switch/1
  Sum3/1 -> Gain1/1
  Gain1/1 -> Transfer Fcn1/1
  Transfer Fcn1/1 -> Transfer Fcn2/1
  Transfer Fcn2/1 -> Transfer Fcn3/1
  Transfer Fcn3/1 -> Saturation/1

== system M4B11_modified_AGC_PI_constant_power/Generator2/Machine Equations  ==
  note: Idg
  note: Iqg
  delta : Inport
  Vgxy : Inport  Port=2
  Ef : Inport  Port=3
  Trip : Inport  Port=4
  Demux : Demux  Outputs=2
  Demux1 : Demux  Outputs=2
  Fcn1 : Fcn  Expr=u(1)*u(3)+u(2)*u(4)
  Fcn2 : Fcn  Expr=(u(3)-u(2))/Xd11
  Fcn3 : Fcn  Expr=(u(1)-u(4))/Xq11
  Fcn4 : Fcn  Expr=u(2)*u(3)-u(1)*u(4)
  Fcn6 : Fcn  Expr=sqrt(u(1)^2+u(2)^2)
  Interface : Subsystem
  Mux1 : Mux  Inputs=2
  Mux2 : Mux  Inputs=2
  Mux3 : Mux  Inputs=2
  Qe : Scope
  Scope{,1..3} (4 alike) : Scope
  Transient Equations : Subsystem
  Pe : Outport
  Igxy1 : Outport  Port=2
  GBxy : Outport  Port=3
  Vg : Outport  Port=4
  wires:
  Fcn3/1 -> Mux3/2
  Fcn2/1 -> Mux3/1
  Mux3/1 -> Demux1/1, Mux2/2, Transient Equations/1(Idqg)
  Interface/1(Vdqg) -> Demux/1, Mux2/1, Fcn6/1, Mux1/1
  Mux1/1 -> Fcn2/1, Fcn3/1
  Mux2/1 -> Fcn1/1, Fcn4/1
  Ef/1 -> Transient Equations/2(Ef)
  Fcn1/1 -> Pe/1
  Fcn6/1 -> Vg/1
  Fcn4/1 -> Qe/1
  delta/1 -> Interface/1(delta)
  Vgxy/1 -> Interface/2(Vgxy)
  Interface/2(Igxy1) -> Igxy1/1
  Interface/3(GBxy) -> GBxy/1
  Transient Equations/1(Eqd'') -> Mux1/2, Interface/3(Eqd'')
  Demux/1 -> Scope1/1
  Demux1/1 -> Scope/1
  Demux/2 -> Scope2/1
  Demux1/2 -> Scope3/1
  Trip/1 -> [Trip]
  [Trip] -> Transient Equations/3(Trip)

== system M4B11_modified_AGC_PI_constant_power/Generator2/Mechanical DE ==
  Pe : Inport
  dPm : Inport  Port=2
  Trip : Inport  Port=3
  Constant1 : Constant  Value=0
  Constant2 : Constant  Value=0
  Gain : Gain  Gain=wB  SaturateOnIntegerOverflow=on  OutDataTypeStr=Inherit: Same as input  ParamDataTypeStr=Inherit: Same as input
  Gain1 : Gain  Gain=1/H  SaturateOnIntegerOverflow=on  OutDataTypeStr=Inherit: Same as input  ParamDataTypeStr=Inherit: Same as input
  Gain2 : Gain  Gain=D  SaturateOnIntegerOverflow=on  OutDataTypeStr=Inherit: Same as input  ParamDataTypeStr=Inherit: Same as input
  Gain5 : Gain  Gain=180/pi  SaturateOnIntegerOverflow=on  OutDataTypeStr=Inherit: Same as input  ParamDataTypeStr=Inherit: Same as input
  Int1 : Integrator  InitialCondition=delta0
  Int2 : Integrator  InitialCondition=w0
  Pm : Constant  Value=Pm0
  Scope2 : Scope
  Scope4 : Scope
  Scope8 : Scope
  Sum2 : Sum  Inputs=-+-+  SaturateOnIntegerOverflow=on
  Sum3 : Sum  Inputs=|+-  SaturateOnIntegerOverflow=on
  Switch{1..4} (4 alike) : Switch  Criteria=u2 ~= 0  Threshold=0.5  InputSameDT=off
  w0 : Constant
  delta : Outport
  w : Outport  Port=2
  wires:
  [Trip] -> Switch3/2, Switch2/2
  Constant1/1 -> Switch3/1, Switch2/1
  Switch3/1 -> Scope4/1, Sum3/1, w/1
  Int2/1 -> Switch3/3
  Switch2/1 -> Int2/1
  Gain1/1 -> Switch2/3
  Trip/1 -> [Trip]
  [Trip] -> Switch1/2, Switch4/2
  Constant2/1 -> Switch4/1, Switch1/1
  Switch4/1 -> delta/1, Scope2/1, Gain5/1
  Int1/1 -> Switch4/3
  Switch1/1 -> Int1/1
  Gain/1 -> Switch1/3
  Gain5/1 -> Scope8/1
  w0/1 -> Sum3/2
  Sum3/1 -> Gain2/1, Gain/1
  Pm/1 -> Sum2/2
  Gain2/1 -> Sum2/1
  Sum2/1 -> Gain1/1
  Pe/1 -> Sum2/3
  dPm/1 -> Sum2/4

== system M4B11_modified_AGC_PI_constant_power/Generator2/Output ==
  Igxy1in : Inport
  GBxyin : Inport  Port=2
  deltain : Inport  Port=3
  Pein : Inport  Port=4
  fin : Inport  Port=5
  Vg : Inport  Port=6
  Bus Creator : BusCreator  Inputs=6
  m : Outport
  Igxy1 : Outport  Port=2
  GBxy : Outport  Port=3
  wires:
  Bus Creator/1 -> m/1
  Igxy1in/1 -> Igxy1/1, Bus Creator/1  "Igxy1"
  GBxyin/1 -> GBxy/1, Bus Creator/2  "GBxy"
  deltain/1 -> Bus Creator/3  "delta"
  Pein/1 -> Bus Creator/4  "Pe"
  fin/1 -> Bus Creator/5  "f"
  Vg/1 -> Bus Creator/6  "Vg"

== system M4B11_modified_AGC_PI_constant_power/Generator2/PSS1 ==
  w : Inport
  Trip : Inport  Port=2
  CT : Constant  Value=0
  Constant : Constant  Value=0
  Gain : Gain  Gain=Kpss  SaturateOnIntegerOverflow=on  OutDataTypeStr=Inherit: Same as input  ParamDataTypeStr=Inherit: Same as input
  Saturation : Saturate  UpperLimit=Upmax  LowerLimit=Upmin
  Sum3 : Sum  Inputs=|+-  SaturateOnIntegerOverflow=on
  Switch : Switch  Threshold=0.5  InputSameDT=off
  Switch1 : Switch  Threshold=0.5  InputSameDT=off
  Transfer Fcn : TransferFcn  Numerator=[Tw_P 0]  Denominator=[Tw_P 1]
  Transfer Fcn1 : TransferFcn  Numerator=[T1_P 1]  Denominator=[T2_P 1]
  Transfer Fcn2 : TransferFcn  Numerator=[T3_P 1]  Denominator=[T4_P 1]
  w0 : Constant
  w1 : Constant  Value=S_PSS
  Upss : Outport
  wires:
  Constant/1 -> Switch1/1
  Trip/1 -> Switch1/2
  Switch1/1 -> Upss/1
  Switch/1 -> Switch1/3
  Transfer Fcn/1 -> Transfer Fcn1/1
  Gain/1 -> Transfer Fcn/1
  w1/1 -> Switch/2
  CT/1 -> Switch/3
  Saturation/1 -> Switch/1
  Sum3/1 -> Gain/1
  Transfer Fcn2/1 -> Saturation/1
  Transfer Fcn1/1 -> Transfer Fcn2/1
  w/1 -> Sum3/1
  w0/1 -> Sum3/2

== system M4B11_modified_AGC_PI_constant_power/Generator3/Excitation System ==
  note: Ef
  Upss : Inport
  Trip : Inport  Port=2
  Vg : Inport  Port=3
  Constant : Constant  Value=0
  KA : Gain  Gain=Ka  SaturateOnIntegerOverflow=on  OutDataTypeStr=Inherit: Same as input  ParamDataTypeStr=Inherit: Same as input
  Saturation : Saturate  UpperLimit=Efmax  LowerLimit=Efmin
  Scope : Scope  NumInputPorts=2
  Sum4 : Sum  Inputs=+-+  SaturateOnIntegerOverflow=on
  Switch : Switch  Criteria=u2 ~= 0  Threshold=0.5  InputSameDT=off
  Vref : Constant  Value=Vref
  Ef : Outport
  wires:
  Trip/1 -> Switch/2
  Constant/1 -> Switch/1
  Switch/1 -> Ef/1
  Saturation/1 -> Switch/3
  Sum4/1 -> KA/1
  KA/1 -> Saturation/1
  Vg/1 -> Sum4/2, Scope/2
  Upss/1 -> Sum4/3
  Vref/1 -> Scope/1, Sum4/1

== system M4B11_modified_AGC_PI_constant_power/Generator3/Governor ==
  w : Inport
  Trip : Inport  Port=2
  CT : Constant  Value=0
  Constant : Constant  Value=0
  Gain1 : Gain  Gain=1/R  SaturateOnIntegerOverflow=on  OutDataTypeStr=Inherit: Same as input  ParamDataTypeStr=Inherit: Same as input
  Saturation : Saturate  UpperLimit=dPmax  LowerLimit=dPmin
  Sum3 : Sum  Inputs=|+-  SaturateOnIntegerOverflow=on
  Switch : Switch  Threshold=0.5  InputSameDT=off
  Switch1 : Switch  Criteria=u2 ~= 0  Threshold=0.5  InputSameDT=off
  Transfer Fcn1 : TransferFcn  Denominator=[Ts_G 1]
  Transfer Fcn2 : TransferFcn  Numerator=[T3_G 1]  Denominator=[Tc_G 1]
  Transfer Fcn3 : TransferFcn  Numerator=[T4_G 1]  Denominator=[T5_G 1]
  w1 : Constant  Value=S_Gov
  wref : Constant
  dPm : Outport
  wires:
  Constant/1 -> Switch1/1
  Switch/1 -> Switch1/3
  Trip/1 -> Switch1/2
  Switch1/1 -> dPm/1
  CT/1 -> Switch/3
  w1/1 -> Switch/2
  wref/1 -> Sum3/1
  w/1 -> Sum3/2
  Saturation/1 -> Switch/1
  Sum3/1 -> Gain1/1
  Gain1/1 -> Transfer Fcn1/1
  Transfer Fcn1/1 -> Transfer Fcn2/1
  Transfer Fcn2/1 -> Transfer Fcn3/1
  Transfer Fcn3/1 -> Saturation/1

== system M4B11_modified_AGC_PI_constant_power/Generator3/Machine Equations  ==
  note: Idg
  note: Iqg
  delta : Inport
  Vgxy : Inport  Port=2
  Ef : Inport  Port=3
  Trip : Inport  Port=4
  Demux : Demux  Outputs=2
  Demux1 : Demux  Outputs=2
  Fcn1 : Fcn  Expr=u(1)*u(3)+u(2)*u(4)
  Fcn2 : Fcn  Expr=(u(3)-u(2))/Xd11
  Fcn3 : Fcn  Expr=(u(1)-u(4))/Xq11
  Fcn4 : Fcn  Expr=u(2)*u(3)-u(1)*u(4)
  Fcn6 : Fcn  Expr=sqrt(u(1)^2+u(2)^2)
  Interface : Subsystem
  Mux1 : Mux  Inputs=2
  Mux2 : Mux  Inputs=2
  Mux3 : Mux  Inputs=2
  Qe : Scope
  Scope{,1..3} (4 alike) : Scope
  Transient Equations : Subsystem
  Pe : Outport
  Igxy1 : Outport  Port=2
  GBxy : Outport  Port=3
  Vg : Outport  Port=4
  wires:
  Fcn3/1 -> Mux3/2
  Fcn2/1 -> Mux3/1
  Mux3/1 -> Demux1/1, Mux2/2, Transient Equations/1(Idqg)
  Interface/1(Vdqg) -> Demux/1, Mux2/1, Fcn6/1, Mux1/1
  Mux1/1 -> Fcn2/1, Fcn3/1
  Mux2/1 -> Fcn1/1, Fcn4/1
  Ef/1 -> Transient Equations/2(Ef)
  Fcn1/1 -> Pe/1
  Fcn6/1 -> Vg/1
  Fcn4/1 -> Qe/1
  delta/1 -> Interface/1(delta)
  Vgxy/1 -> Interface/2(Vgxy)
  Interface/2(Igxy1) -> Igxy1/1
  Interface/3(GBxy) -> GBxy/1
  Transient Equations/1(Eqd'') -> Mux1/2, Interface/3(Eqd'')
  Demux/1 -> Scope1/1
  Demux1/1 -> Scope/1
  Demux/2 -> Scope2/1
  Demux1/2 -> Scope3/1
  Trip/1 -> [Trip]
  [Trip] -> Transient Equations/3(Trip)

== system M4B11_modified_AGC_PI_constant_power/Generator3/Mechanical DE ==
  Pe : Inport
  dPm : Inport  Port=2
  Trip : Inport  Port=3
  Constant1 : Constant  Value=0
  Constant2 : Constant  Value=0
  Gain : Gain  Gain=wB  SaturateOnIntegerOverflow=on  OutDataTypeStr=Inherit: Same as input  ParamDataTypeStr=Inherit: Same as input
  Gain1 : Gain  Gain=1/H  SaturateOnIntegerOverflow=on  OutDataTypeStr=Inherit: Same as input  ParamDataTypeStr=Inherit: Same as input
  Gain2 : Gain  Gain=D  SaturateOnIntegerOverflow=on  OutDataTypeStr=Inherit: Same as input  ParamDataTypeStr=Inherit: Same as input
  Gain5 : Gain  Gain=180/pi  SaturateOnIntegerOverflow=on  OutDataTypeStr=Inherit: Same as input  ParamDataTypeStr=Inherit: Same as input
  Int1 : Integrator  InitialCondition=delta0
  Int2 : Integrator  InitialCondition=w0
  Pm : Constant  Value=Pm0
  Scope2 : Scope
  Scope4 : Scope
  Scope8 : Scope
  Sum2 : Sum  Inputs=-+-+  SaturateOnIntegerOverflow=on
  Sum3 : Sum  Inputs=|+-  SaturateOnIntegerOverflow=on
  Switch{1..4} (4 alike) : Switch  Criteria=u2 ~= 0  Threshold=0.5  InputSameDT=off
  w0 : Constant
  delta : Outport
  w : Outport  Port=2
  wires:
  [Trip] -> Switch3/2, Switch2/2
  Constant1/1 -> Switch3/1, Switch2/1
  Switch3/1 -> Scope4/1, Sum3/1, w/1
  Int2/1 -> Switch3/3
  Switch2/1 -> Int2/1
  Gain1/1 -> Switch2/3
  Trip/1 -> [Trip]
  [Trip] -> Switch1/2, Switch4/2
  Constant2/1 -> Switch4/1, Switch1/1
  Switch4/1 -> delta/1, Scope2/1, Gain5/1
  Int1/1 -> Switch4/3
  Switch1/1 -> Int1/1
  Gain/1 -> Switch1/3
  Gain5/1 -> Scope8/1
  w0/1 -> Sum3/2
  Sum3/1 -> Gain2/1, Gain/1
  Pm/1 -> Sum2/2
  Gain2/1 -> Sum2/1
  Sum2/1 -> Gain1/1
  Pe/1 -> Sum2/3
  dPm/1 -> Sum2/4

== system M4B11_modified_AGC_PI_constant_power/Generator3/Output ==
  Igxy1in : Inport
  GBxyin : Inport  Port=2
  deltain : Inport  Port=3
  Pein : Inport  Port=4
  fin : Inport  Port=5
  Vg : Inport  Port=6
  Bus Creator : BusCreator  Inputs=6
  m : Outport
  Igxy1 : Outport  Port=2
  GBxy : Outport  Port=3
  wires:
  Bus Creator/1 -> m/1
  Igxy1in/1 -> Igxy1/1, Bus Creator/1  "Igxy1"
  GBxyin/1 -> GBxy/1, Bus Creator/2  "GBxy"
  deltain/1 -> Bus Creator/3  "delta"
  Pein/1 -> Bus Creator/4  "Pe"
  fin/1 -> Bus Creator/5  "f"
  Vg/1 -> Bus Creator/6  "Vg"

== system M4B11_modified_AGC_PI_constant_power/Generator3/PSS1 ==
  w : Inport
  Trip : Inport  Port=2
  CT : Constant  Value=0
  Constant : Constant  Value=0
  Gain : Gain  Gain=Kpss  SaturateOnIntegerOverflow=on  OutDataTypeStr=Inherit: Same as input  ParamDataTypeStr=Inherit: Same as input
  Saturation : Saturate  UpperLimit=Upmax  LowerLimit=Upmin
  Sum3 : Sum  Inputs=|+-  SaturateOnIntegerOverflow=on
  Switch : Switch  Threshold=0.5  InputSameDT=off
  Switch1 : Switch  Threshold=0.5  InputSameDT=off
  Transfer Fcn : TransferFcn  Numerator=[Tw_P 0]  Denominator=[Tw_P 1]
  Transfer Fcn1 : TransferFcn  Numerator=[T1_P 1]  Denominator=[T2_P 1]
  Transfer Fcn2 : TransferFcn  Numerator=[T3_P 1]  Denominator=[T4_P 1]
  w0 : Constant
  w1 : Constant  Value=S_PSS
  Upss : Outport
  wires:
  Constant/1 -> Switch1/1
  Trip/1 -> Switch1/2
  Switch1/1 -> Upss/1
  Switch/1 -> Switch1/3
  Transfer Fcn/1 -> Transfer Fcn1/1
  Gain/1 -> Transfer Fcn/1
  w1/1 -> Switch/2
  CT/1 -> Switch/3
  Saturation/1 -> Switch/1
  Sum3/1 -> Gain/1
  Transfer Fcn2/1 -> Saturation/1
  Transfer Fcn1/1 -> Transfer Fcn2/1
  w/1 -> Sum3/1
  w0/1 -> Sum3/2

== system M4B11_modified_AGC_PI_constant_power/Wind Generator - DFIG1/Asynchronous Machine Equations  ==
  note: Vsdq
  s / ω_B : Inport
  Vgxy : Inport  Port=2
  Vrxy : Inport  Port=3
  "Trip " : Inport  Port=4
  3th order Transient Equations : Subsystem
  Add : Sum  Inputs=+-
  Constant : Constant  Value=Za
  Constant1 : Constant  Value=0
  Fcn6 : Fcn  Expr=sqrt(u(1)^2+u(2)^2)
  Gain2 : Gain  Gain=NPf
  Interface : Subsystem
  Multiply : Product  Multiplication=Matrix(*)
  Mux2 : Mux  Inputs=2
  Mux4 : Mux  Inputs=2
  Ps_ : Fcn  Expr=u(1)*u(3)+u(2)*u(4)
  Qs_ : Fcn  Expr=u(2)*u(3)-u(1)*u(4)
  Scope : Scope
  Scope1 : Scope
  Selector : Selector  InputPortWidth=2  IndexOptions=Index vector (dialog)  Indices=[2 1]  OutputSizes=1
  Te_ : Fcn  Expr=u(2)*u(3)+u(1)*u(4)
  Te : Outport
  Ps : Outport  Port=2
  Qs : Outport  Port=3
  Irxy : Outport  Port=4
  Exy : Outport  Port=5
  Isxy1 : Outport  Port=6
  GBxy : Outport  Port=7
  wires:
  "Trip "/1 -> 3th order Transient Equations/4(Trip)
  3th order Transient Equations/1(Irxy) -> Irxy/1
  Qs_/1 -> Qs/1, Scope/1
  Constant1/1 -> Interface/1(delta)
  Gain2/1 -> Te/1
  Vgxy/1 -> Add/1, Fcn6/1, Mux2/1
  Add/1 -> Multiply/2
  Constant/1 -> Multiply/1
  Selector/1 -> Exy/1, Add/2
  Te_/1 -> Gain2/1
  Mux4/1 -> Te_/1
  s / ω_B/1 -> 3th order Transient Equations/3(s / ω_B)
  Ps_/1 -> Ps/1
  Interface/1(Igxy1) -> Isxy1/1
  Interface/2(GBxy) -> GBxy/1
  Mux2/1 -> Qs_/1, Ps_/1
  Vrxy/1 -> 3th order Transient Equations/2(Vrxy)
  Multiply/1 -> 3th order Transient Equations/1(Isxy), Mux4/1, Mux2/2
  Fcn6/1 -> Scope1/1
  3th order Transient Equations/2(Eyx) -> Mux4/2, Selector/1, Interface/2(Eqd)

== system M4B11_modified_AGC_PI_constant_power/Wind Generator - DFIG1/Converter function ==
  Vsxy : Inport
  Vcxy : Inport  Port=2
  Trip : Inport  Port=3
  Change_choke : Gain  Gain=[1 -1]  SaturateOnIntegerOverflow=on  OutDataTypeStr=Inherit: Same as input  ParamDataTypeStr=Inherit: Same as input
  Constant2 : Constant  Value=0
  GSC_Idq : Integrator  InitialCondition=[Icx0 Icy0]
  L_choke : Gain  Gain=Lg  SaturateOnIntegerOverflow=on  OutDataTypeStr=Inherit: Same as input  ParamDataTypeStr=Inherit: Same as input
  R_choke : Gain  Gain=Rg  SaturateOnIntegerOverflow=on  OutDataTypeStr=Inherit: Same as input  ParamDataTypeStr=Inherit: Same as input
  Selector : Selector  InputPortWidth=2  IndexOptions=Index vector (dialog)  Indices=[2 1]  OutputSizes=1
  Sum : Sum  Inputs=+--+  SaturateOnIntegerOverflow=on
  Switch1 : Switch  Criteria=u2 ~= 0  Threshold=0.5  InputSameDT=off
  Switch4 : Switch  Criteria=u2 ~= 0  Threshold=0.5  InputSameDT=off
  W/L : Gain  Gain=wB / Lg  SaturateOnIntegerOverflow=on  OutDataTypeStr=Inherit: Same as input  ParamDataTypeStr=Inherit: Same as input
  Ixy_gsc : Outport
  wires:
  Switch4/1 -> Ixy_gsc/1, R_choke/1, Selector/1
  GSC_Idq/1 -> Switch4/3
  Switch1/1 -> GSC_Idq/1
  W/L/1 -> Switch1/3
  Constant2/1 -> Switch4/1, Switch1/1
  Trip/1 -> Switch1/2, Switch4/2
  Vcxy/1 -> Sum/2
  Change_choke/1 -> Sum/4
  Sum/1 -> W/L/1
  R_choke/1 -> Sum/3
  Vsxy/1 -> Sum/1
  Selector/1 -> L_choke/1
  L_choke/1 -> Change_choke/1
